simulink model "FOC_physical_2_Testing_mathmatical"  (R2024b)
settings: Solver=FixedStepAuto  StartTime=0.0  StopTime=4  FixedStep=1e-5  RelTol=1e-3
undefined symbols (not defined in the file): B, DiscIntNeverNeededParam, Down, dspblkCoreblockFVToolHelper, gcbh, GPTRIP1SEL, J, Ki_current, Ki_q, Ki_s, Ki_speed, Kp_current, Kp_q, Kp_s, Kp_speed, lambda, lamdaM, Ld, Ls, ma, P, Rs, T_max, T_period, Tc, TZ1, Up, Vdc
libraries: simulink x12, c2802xlib x7, spsIGBTDiodeLib x6, spsCurrentMeasurementLib x3, eeStairGenerator x2, spsStairGeneratorLib x2, spsDCVoltageSourceLib x1, spsPermanentMagnetSynchronousMachineLib x1, eeGeneralControl x1, mcbpositiondecoderlib x1, c280xlib x1, spspowerguiLib x1
(part 3 of 3)

== system FOC_physical_2_Testing_mathmatical/Subsystem3/voltage limits by maintaining the same ration/Voltage_to_be_Limited ==
  Vq_ref_new : Inport
  Vd_ref_new : Inport  Port=2
  Action Port : ActionPort  ActionPortLabel=else
  Divide1 : Product  Inputs=*/  OutDataTypeStr=single
  Divide2 : Product  Inputs=/*  OutDataTypeStr=single
  Gain : Gain  Gain=sqrt(3)
  Gain1 : Gain  Gain=Vdc * ma
  Gain2 : Gain  Gain=Vdc * ma
  Square : Math  Operator=square  OutDataTypeStr=single
  Square Root : Sqrt  OutDataTypeStr=single  IntermediateResultsDataTypeStr=single
  Square1 : Math  Operator=square  OutDataTypeStr=single
  Sum : Sum  OutDataTypeStr=single  AccumDataTypeStr=single
  Vq_ref_2 : Outport
  Vd_ref_2 : Outport  Port=2
  wires:
  Vq_ref_new/1 -> Gain1/1, Square/1
  Sum/1 -> Square Root/1
  Vd_ref_new/1 -> Square1/1, Gain2/1
  Square1/1 -> Sum/2
  Square/1 -> Sum/1
  Divide1/1 -> Vq_ref_2/1
  Square Root/1 -> Gain/1
  Divide2/1 -> Vd_ref_2/1
  Gain/1 -> Divide2/1, Divide1/2
  Gain1/1 -> Divide1/1
  Gain2/1 -> Divide2/2

== system FOC_physical_2_Testing_mathmatical/Subsystem/SVPWM/Subsystem1/Theta dash ==
  Sector : Inport
  angle : Inport  Port=2
  Constant : Constant
  Display : Display
  Gain : Gain  Gain=(pi/3)
  Subtract : Sum  Inputs=-+
  Subtract1 : Sum  Inputs=-+
  Theta dash : Outport
  wires:
  angle/1 -> Subtract/2
  Gain/1 -> Subtract/1
  Constant/1 -> Subtract1/1
  Sector/1 -> Subtract1/2
  Subtract1/1 -> Gain/1
  Subtract/1 -> Display/1, Theta dash/1

== system FOC_physical_2_Testing_mathmatical/Subsystem/Subsystem/Park and Clark transformation1/Subsystem ==
  In1 : Inport
  In2 : Inport  Port=2
  In3 : Inport  Port=3
  Add : Sum  Inputs=+--
  Add1 : Sum  Inputs=+-
  Gain : Gain  Gain=2/3
  Gain1 : Gain  Gain=1/2
  Gain2 : Gain  Gain=1/2
  Gain3 : Gain  Gain=sqrt(3)/2
  Gain4 : Gain  Gain=sqrt(3)/2
  Gain5 : Gain  Gain=2/3
  Valpha : Outport
  Vbeta : Outport  Port=2
  wires:
  In1/1 -> Add/1
  Gain/1 -> Valpha/1
  Add1/1 -> Gain5/1
  Add/1 -> Gain/1
  In3/1 -> Gain4/1, Gain1/1
  Gain4/1 -> Add1/2
  Gain5/1 -> Vbeta/1
  In2/1 -> Gain3/1, Gain2/1
  Gain2/1 -> Add/2
  Gain1/1 -> Add/3
  Gain3/1 -> Add1/1

== system FOC_physical_2_Testing_mathmatical/Subsystem/Subsystem/Park and Clark transformation1/Subsystem1 ==
  Theta : Inport
  Valpha : Inport  Port=2
  Vbeta : Inport  Port=3
  Add : Sum
  Add1 : Sum
  Cos : Trigonometry  Operator=cos
  Cos1 : Trigonometry  Operator=cos
  Gain : Gain  Gain=-1
  Product{,1..3} (4 alike) : Product
  Sin : Trigonometry
  Sin1 : Trigonometry
  Vd : Outport
  Vq : Outport  Port=2
  wires:
  Add1/1 -> Vq/1
  Valpha/1 -> Product/2, [Valpha]
  Add/1 -> Vd/1
  [Valpha] -> Product3/1
  Vbeta/1 -> Product1/2, Product2/1
  Product2/1 -> Add1/1
  Product3/1 -> Add1/2
  Cos/1 -> Product/1
  Cos1/1 -> Product2/2
  [Theta] -> Cos1/1, Sin1/1
  Product1/1 -> Add/1
  Theta/1 -> Sin/1, Cos/1, [Theta]
  Sin/1 -> Product1/1
  Product/1 -> Add/2
  Gain/1 -> Product3/2
  Sin1/1 -> Gain/1

== system FOC_physical_2_Testing_mathmatical/Subsystem3/SVPWM/Subsystem1/Theta dash ==
  Sector : Inport
  angle : Inport  Port=2
  Constant : Constant
  Display : Display
  Gain : Gain  Gain=(pi/3)
  Subtract : Sum  Inputs=-+
  Subtract1 : Sum  Inputs=-+
  Theta dash : Outport
  wires:
  angle/1 -> Subtract/2
  Gain/1 -> Subtract/1
  Constant/1 -> Subtract1/1
  Sector/1 -> Subtract1/2
  Subtract1/1 -> Gain/1
  Subtract/1 -> Display/1, Theta dash/1

== system FOC_physical_2_Testing_mathmatical/Subsystem3/Subsystem/Park and Clark transformation1/Subsystem ==
  In1 : Inport
  In2 : Inport  Port=2
  In3 : Inport  Port=3
  Add : Sum  Inputs=+--
  Add1 : Sum  Inputs=+-
  Gain : Gain  Gain=2/3
  Gain1 : Gain  Gain=1/2
  Gain2 : Gain  Gain=1/2
  Gain3 : Gain  Gain=sqrt(3)/2
  Gain4 : Gain  Gain=sqrt(3)/2
  Gain5 : Gain  Gain=2/3
  Valpha : Outport
  Vbeta : Outport  Port=2
  wires:
  In1/1 -> Add/1
  Gain/1 -> Valpha/1
  Add1/1 -> Gain5/1
  Add/1 -> Gain/1
  In3/1 -> Gain4/1, Gain1/1
  Gain4/1 -> Add1/2
  Gain5/1 -> Vbeta/1
  In2/1 -> Gain3/1, Gain2/1
  Gain2/1 -> Add/2
  Gain1/1 -> Add/3
  Gain3/1 -> Add1/1

== system FOC_physical_2_Testing_mathmatical/Subsystem3/Subsystem/Park and Clark transformation1/Subsystem1 ==
  Theta : Inport
  Valpha : Inport  Port=2
  Vbeta : Inport  Port=3
  Add : Sum
  Add1 : Sum
  Cos : Trigonometry  Operator=cos
  Cos1 : Trigonometry  Operator=cos
  Gain : Gain  Gain=-1
  Product{,1..3} (4 alike) : Product
  Sin : Trigonometry
  Sin1 : Trigonometry
  Vd : Outport
  Vq : Outport  Port=2
  wires:
  Add1/1 -> Vq/1
  Valpha/1 -> Product/2, [Valpha]
  Add/1 -> Vd/1
  [Valpha] -> Product3/1
  Vbeta/1 -> Product1/2, Product2/1
  Product2/1 -> Add1/1
  Product3/1 -> Add1/2
  Cos/1 -> Product/1
  Cos1/1 -> Product2/2
  [Theta] -> Cos1/1, Sin1/1
  Product1/1 -> Add/1
  Theta/1 -> Sin/1, Cos/1, [Theta]
  Sin/1 -> Product1/1
  Product/1 -> Add/2
  Gain/1 -> Product3/2
  Sin1/1 -> Gain/1

== matlab function FOC_physical_2_Testing_mathmatical/Subsystem/SVPWM/Subsystem2/MATLAB Function ==
  data: TS1 output; u input; TS3 output; TS5 output; v input; w input; g input; S input
function [TS1, TS3,TS5] = fcn(u, v, w, g,S)

switch S
    case 1
        TS1 = u;
        TS3 = v;
        TS5 = w;
    case 2
        TS1 = g;
        TS3 = u;
        TS5 = w;
    case 3
        TS1 = w;
        TS3 = u;
        TS5 = v;
    case 4
        TS1 = w;
        TS3 = g;
        TS5 = u;
    case 5
        TS1 = v;
        TS3 = w;
        TS5 = u;
    case 6
        TS1 = u;
        TS3 = w;
        TS5 = g;
    otherwise
      TS1=0;  
      TS3=0;  
      TS5=0; 
end
end

== matlab function FOC_physical_2_Testing_mathmatical/Subsystem/SVPWM/Sector detection ==
  data: u input; S output
function S = fcn(u)

u = (180/pi)* u;

if(u < 60 && u >= 0)
    u = 1;
elseif(u < 120 && u >= 60)
    u = 2;
elseif(u < 180 && u >= 120)
    u = 3;
elseif(u < -120 && u >= -180)
u = 4;
elseif(u < -60 && u >= -120)
u = 5;
elseif(u < 0 && u >= -60)
u = 6;
else
    u = 0;
end
S = u;

== matlab function FOC_physical_2_Testing_mathmatical/SVPWM Technique/Sector Detector ==
  data: u input; S output
function S = fcn(u)

  u= 180/(pi)*u ; % rad to degree
  
if (u>=0)&&(u<60)
  u = 1  ; 
elseif (u>=60)&&(u<120)
  u = 2  ;  
elseif (u>=120)&&(u<180)
  u = 3  ;  
elseif (u>=-180)&&(u<-120)
  u = 4  ;
elseif (u>=-120)&&(u<-60)
  u = 5  ;
elseif (u>=-60)&&(u<0)
  u = 6  ;
else
  u=0 ; 
end

S = u;

== matlab function FOC_physical_2_Testing_mathmatical/SVPWM Technique/Step 3- Determine the switching time of each transistor (S1 to S6) /Sector detection1 ==
  data: s input; u input; Ts1 output; Ts3 output; v input; w input; g input; Ts5 output
function [Ts1,Ts3,Ts5] = fcn(s,u,v,w,g)

switch s 
  
 case 1 
  Ts1 = u ; 
  Ts3 = v ;
  Ts5 = w ;
 case 2 
  Ts1 = g ; 
  Ts3 = u ; 
  Ts5 = w ;
 case 3 
  Ts1 = w ;
  Ts3 = u ; 
  Ts5 = v ; 
 case 4 
  Ts1 = w ;
  Ts3 = g ; 
  Ts5 = u ;
 case 5 
  Ts1 = v ;
  Ts3 = w ; 
  Ts5 = u ;
 case 6 
  Ts1 = u ;
  Ts3 = w ; 
  Ts5 = g ;
 otherwise 
 Ts1 = 0 ; 
 Ts3 = 0 ;
 Ts5 = 0 ;
 end 

end

== matlab function FOC_physical_2_Testing_mathmatical/Subsystem3/SVPWM/Sector detection ==
  data: u input; S output
function S = fcn(u)

u = (180/pi)* u;

if(u < 60 && u >= 0)
    u = 1;
elseif(u < 120 && u >= 60)
    u = 2;
elseif(u < 180 && u >= 120)
    u = 3;
elseif(u < -120 && u >= -180)
u = 4;
elseif(u < -60 && u >= -120)
u = 5;
elseif(u < 0 && u >= -60)
u = 6;
else
    u = 0;
end
S = u;

== matlab function FOC_physical_2_Testing_mathmatical/Subsystem3/SVPWM/Subsystem2/MATLAB Function ==
  data: TS1 output; u input; TS3 output; TS5 output; v input; w input; g input; S input
function [TS1, TS3,TS5] = fcn(u, v, w, g,S)

switch S
    case 1
        TS1 = u;
        TS3 = v;
        TS5 = w;
    case 2
        TS1 = g;
        TS3 = u;
        TS5 = w;
    case 3
        TS1 = w;
        TS3 = u;
        TS5 = v;
    case 4
        TS1 = w;
        TS3 = g;
        TS5 = u;
    case 5
        TS1 = v;
        TS3 = w;
        TS5 = u;
    case 6
        TS1 = u;
        TS3 = w;
        TS5 = g;
    otherwise
      TS1=0;  
      TS3=0;  
      TS5=0; 
end
end
